simulink model "ex1_2"  (R2020a)
settings: Solver=VariableStepAuto  StartTime=0.0  StopTime=4  MaxStep=1e-6  RelTol=1e-3
settings Model: Creator=반달  LastModifiedBy=반달
settings SolverCC: ZeroCrossAlgorithm=Adaptive

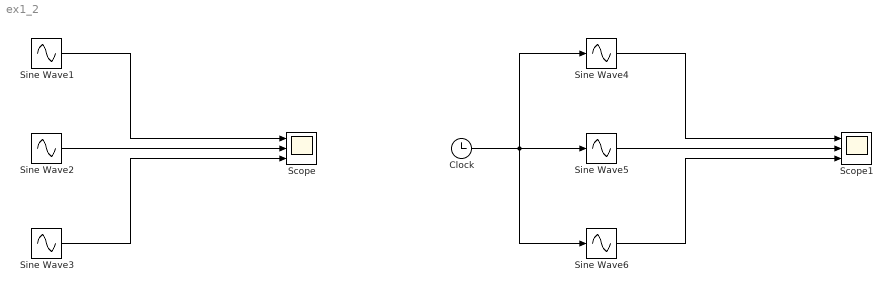
== system ex1_2 ==
  Clock : Clock
  Scope : Scope  NumInputPorts=3
  Scope1 : Scope  NumInputPorts=3
  Sine Wave1 : Sin  Amplitude=2  Frequency=2*pi  SampleTime=0
  Sine Wave2 : Sin  Frequency=2*pi  Phase=pi/2  SampleTime=0
  Sine Wave3 : Sin  Amplitude=0.5  Frequency=2*pi*2  SampleTime=0
  Sine Wave4 : Sin  TimeSource=Use external signal  Amplitude=2  Frequency=2*pi  SampleTime=0
  Sine Wave5 : Sin  TimeSource=Use external signal  Frequency=2*pi  Phase=pi/2  SampleTime=0
  Sine Wave6 : Sin  TimeSource=Use external signal  Amplitude=0.5  Frequency=2*pi*2  SampleTime=0
  wires:
  Sine Wave1/1 -> Scope/1
  Sine Wave2/1 -> Scope/2
  Sine Wave3/1 -> Scope/3
  Sine Wave4/1 -> Scope1/1
  Sine Wave6/1 -> Scope1/3
  Sine Wave5/1 -> Scope1/2
  Clock/1 -> Sine Wave5/1, Sine Wave6/1, Sine Wave4/1
